simulink model "flightController"  (R2017a)
settings: Solver=ode3  StartTime=0  StopTime=10.0  FixedStep=Ts  RelTol=1e-3  EnableMultiTasking=on
undefined symbols (not defined in the file): Controller, DiscIntNeverNeededParam, Ts, Vehicle
settings Model: Creator=The MathWorks, Inc.  LastModifiedBy=Santy
settings DataIOCC: LimitDataPoints=on  SaveFormat=Array
settings OptimizationCC: BlockReduction=off  DefaultParameterBehavior=Inlined  BufferReuse=off  PassReuseOutputArgsThreshold=0
settings DebuggingCC: AlgebraicLoopMsg=none  ParameterPrecisionLossMsg=none  ParameterTunabilityLossMsg=error  UnconnectedInputMsg=none  UnconnectedOutputMsg=none  UnconnectedLineMsg=none  BusObjectLabelMismatch=error  SFUnexpectedBacktrackingDiag=warning  SFNoUnconditionalDefaultTransitionDiag=warning  SFExecutionAtInitializationDiag=none
settings ModelReferenceCC: ModelReferenceNumInstancesAllowed=Single  PropagateSignalLabelsOutOfModel=off
settings RTWCC: GenCodeOnly=on  TemplateMakefile=RTW.MSVCBuild  Description=Create Visual C/C++ Solution File for Simulink Coder  GenerateReport=on  LaunchReport=on
settings CodeAppCC: ForceParamTrailComments=on  MaxIdLength=63  OperatorAnnotations=on  MATLABSourceComments=on
settings GRTTargetCC: TargetLangStandard=C89/C90 (ANSI)
settings ConfigComp: CovMetricSettings=dw  CovHtmlReporting=on  CovSaveCumulativeToWorkspaceVar=on  CovSaveSingleToWorkspaceVar=on  CovExternalEMLEnable=off  CovSFcnEnable=off

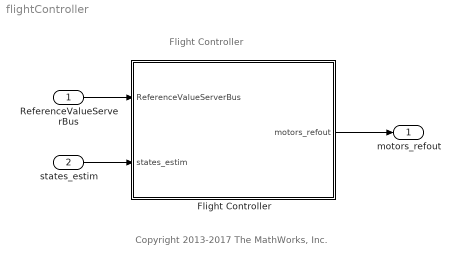
== system flightController ==
  note: Flight Controller
  note: Copyright 2013-2017 The MathWorks, Inc.
  ReferenceValueServerBus : Inport  OutDataTypeStr=Bus: CommandBus  BusOutputAsStruct=on
  states_estim : Inport  Port=2  OutDataTypeStr=Bus: statesEstim_t  BusOutputAsStruct=on
  Flight Controller : Subsystem
  motors_refout : Outport
  wires:
  ReferenceValueServerBus/1 -> Flight Controller/1(ReferenceValueServerBus)
  states_estim/1 -> Flight Controller/2(states_estim)
  Flight Controller/1(motors_refout) -> motors_refout/1

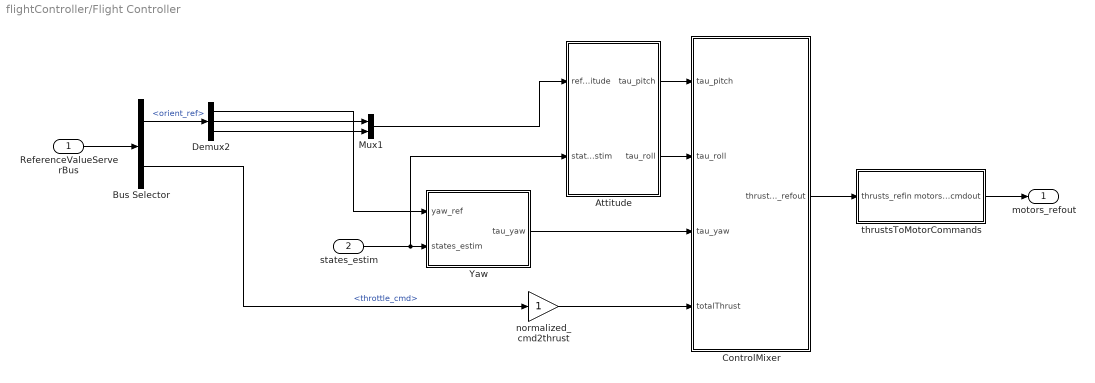
== system flightController/Flight Controller ==
  ReferenceValueServerBus : Inport
  states_estim : Inport  Port=2
  Attitude : Subsystem
  Bus Selector : BusSelector  OutputSignals=orient_ref,throttle_cmd
  ControlMixer : Subsystem
  Demux2 : Demux  Outputs=3
  Mux1 : Mux  Inputs=2
  Yaw : Subsystem
  normalized_cmd2thrust : Gain
  thrustsToMotorCommands : Subsystem
  motors_refout : Outport
  wires:
  Demux2/3 -> Mux1/2
  thrustsToMotorCommands/1(motors_cmdout) -> motors_refout/1
  ReferenceValueServerBus/1 -> Bus Selector/1
  Bus Selector/1 -> Demux2/1  "<orient_ref>"
  Demux2/1 -> Yaw/1(yaw_ref)
  Demux2/2 -> Mux1/1
  ControlMixer/1(thrusts_refout) -> thrustsToMotorCommands/1(thrusts_refin)
  states_estim/1 -> Attitude/2(states_estim), Yaw/2(states_estim)
  Attitude/1(tau_pitch) -> ControlMixer/1(tau_pitch)
  Attitude/2(tau_roll) -> ControlMixer/2(tau_roll)
  Yaw/1(tau_yaw) -> ControlMixer/3(tau_yaw)
  Mux1/1 -> Attitude/1(refAttitude)
  Bus Selector/2 -> normalized_cmd2thrust/1  "<throttle_cmd>"
  normalized_cmd2thrust/1 -> ControlMixer/4(totalThrust)

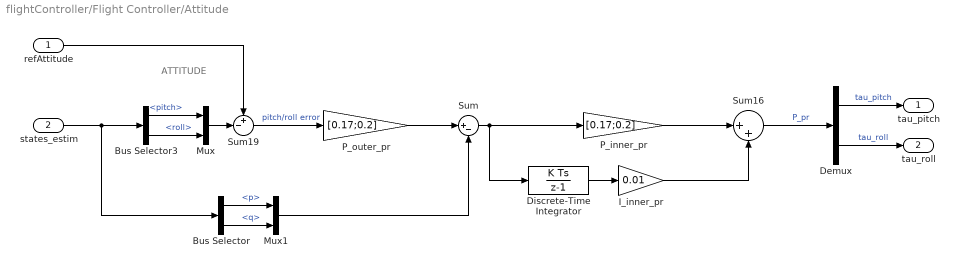
== system flightController/Flight Controller/Attitude ==
  note: ATTITUDE
  refAttitude : Inport
  states_estim : Inport  Port=2
  Bus Selector : BusSelector  OutputSignals=p,q
  Bus Selector3 : BusSelector  OutputSignals=pitch,roll
  Demux : Demux  Outputs=2
  Discrete-Time Integrator : DiscreteIntegrator  InitialConditionSetting=State (most efficient)  SampleTime=Ts  LimitOutput=on  UpperSaturationLimit=2  LowerSaturationLimit=-2  ICPrevOutput=DiscIntNeverNeededParam  ICPrevScaledInput=DiscIntNeverNeededParam
  I_inner_pr : Gain  Gain=0.01
  Mux : Mux  Inputs=2
  Mux1 : Mux  Inputs=2
  P_inner_pr : Gain  Gain=[0.17;0.2]
  P_outer_pr : Gain  Gain=[0.17;0.2]
  Sum : Sum  Inputs=|+-
  Sum16 : Sum  Inputs=|++  AccumDataTypeStr=single  OutDataTypeStr=single  SaturateOnIntegerOverflow=on
  Sum19 : Sum  Inputs=+-|
  tau_pitch : Outport
  tau_roll : Outport  Port=2
  wires:
  Sum16/1 -> Demux/1  "P_pr"
  Bus Selector3/1 -> Mux/1  "<pitch>"
  I_inner_pr/1 -> Sum16/2
  Sum19/1 -> P_outer_pr/1  "pitch/roll error"
  Discrete-Time Integrator/1 -> I_inner_pr/1
  Demux/1 -> tau_pitch/1  "tau_pitch"
  Demux/2 -> tau_roll/1  "tau_roll"
  states_estim/1 -> Bus Selector/1, Bus Selector3/1
  refAttitude/1 -> Sum19/1
  Mux/1 -> Sum19/2
  Bus Selector3/2 -> Mux/2  "<roll>"
  Bus Selector/1 -> Mux1/1  "<p>"
  Bus Selector/2 -> Mux1/2  "<q>"
  Mux1/1 -> Sum/2
  P_outer_pr/1 -> Sum/1
  Sum/1 -> Discrete-Time Integrator/1, P_inner_pr/1
  P_inner_pr/1 -> Sum16/1

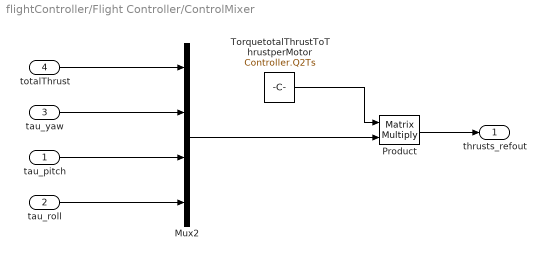
== system flightController/Flight Controller/ControlMixer ==
  tau_pitch : Inport
  tau_roll : Inport  Port=2
  tau_yaw : Inport  Port=3
  totalThrust : Inport  Port=4
  Mux2 : Mux
  Product : Product  Multiplication=Matrix(*)  RndMeth=Zero
  TorquetotalThrustToThrustperMotor : Constant  Value=Controller.Q2Ts  OutDataTypeStr=single
  thrusts_refout : Outport
  wires:
  Product/1 -> thrusts_refout/1
  tau_roll/1 -> Mux2/4
  tau_pitch/1 -> Mux2/3
  tau_yaw/1 -> Mux2/2
  totalThrust/1 -> Mux2/1
  TorquetotalThrustToThrustperMotor/1 -> Product/1
  Mux2/1 -> Product/2

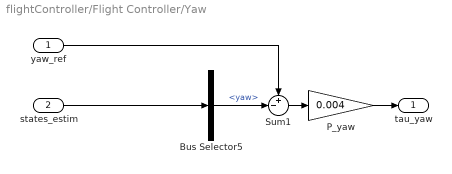
== system flightController/Flight Controller/Yaw ==
  yaw_ref : Inport
  states_estim : Inport  Port=2
  Bus Selector5 : BusSelector  OutputSignals=yaw
  P_yaw : Gain  Gain=0.004  ParamDataTypeStr=single  OutDataTypeStr=single
  Sum1 : Sum  Inputs=+-|  AccumDataTypeStr=single  OutDataTypeStr=single  SaturateOnIntegerOverflow=on
  tau_yaw : Outport
  wires:
  Sum1/1 -> P_yaw/1
  states_estim/1 -> Bus Selector5/1
  P_yaw/1 -> tau_yaw/1
  Bus Selector5/1 -> Sum1/2  "<yaw>"
  yaw_ref/1 -> Sum1/1

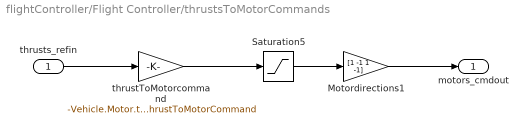
== system flightController/Flight Controller/thrustsToMotorCommands ==
  thrusts_refin : Inport
  Motordirections1 : Gain  Gain=[1 -1 1 -1]
  Saturation5 : Saturate  UpperLimit=Vehicle.Motor.maxLimit  LowerLimit=Vehicle.Motor.minLimit
  thrustToMotorcommand : Gain  Gain=-Vehicle.Motor.thrustToMotorCommand
  motors_cmdout : Outport
  wires:
  Saturation5/1 -> Motordirections1/1
  Motordirections1/1 -> motors_cmdout/1
  thrustToMotorcommand/1 -> Saturation5/1
  thrusts_refin/1 -> thrustToMotorcommand/1
